simulink model "systema"  (Simulink 8.2)
settings: Solver=ode4  StartTime=0.0  StopTime=20  FixedStep=0.01  RelTol=1e-3
CloseFcn:
  | rtwprivate ssgencode ModelCloseRequest systema
settings Model: Creator=Administrator  LastModifiedBy=adnanmartini  BufferReuse=off
settings DataIOCC: SignalLoggingName=sigsOut
settings OptimizationCC: OptimizeBlockIOStorage=off  BufferReuse=off  ExpressionFolding=off  ExpressionDepthLimit=128  FoldNonRolledExpr=off  LocalBlockOutputs=off  InitFltsAndDblsToZero=on
settings DebuggingCC: SaveWithParameterizedLinksMsg=none  SignalResolutionControl=TryResolveAllWithWarning  SolverPrmCheckMsg=none  MultiTaskDSMMsg=warning  MultiTaskCondExecSysMsg=none
settings HardwareCC: TargetUnknown=on
settings SFSimCC: SimParseCustomCode=off
settings RTWCC: IncludeERTFirstTime=on
settings CodeAppCC: IgnoreCustomStorageClasses=off
settings GRTTargetCC: TargetFcnLib=ansi_tfl_tmw.mat  ModelReferenceCompliant=off  MatFileLogging=off

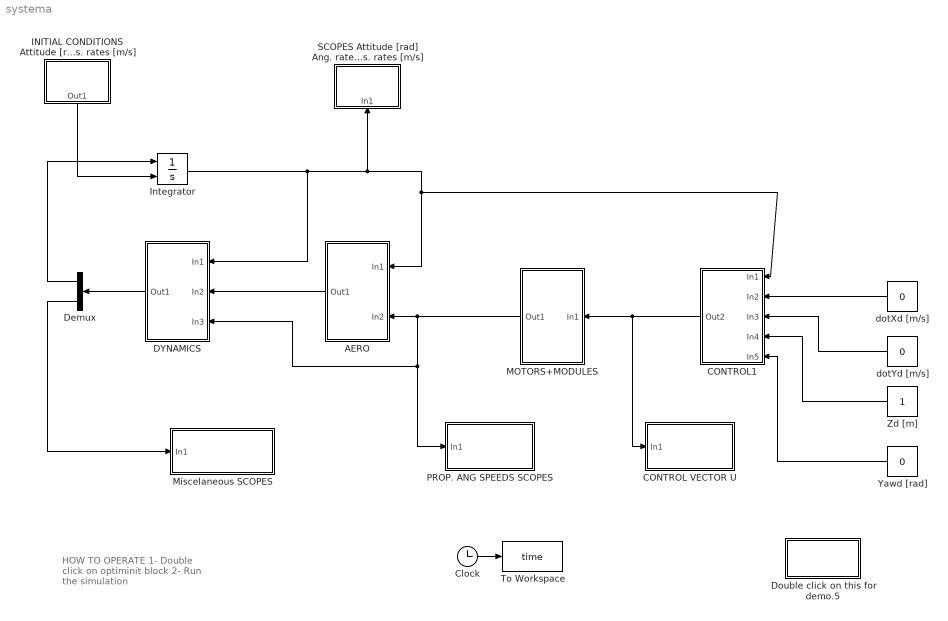
== system systema ==
  note: HOW TO OPERATE
      | 1- Double click on optiminit block
      | 2- Run the simulation
  AERO : Subsystem
  CONTROL VECTOR U : Subsystem
  CONTROL1 : Subsystem
  Clock : Clock
  DYNAMICS : Subsystem
  Demux : Demux  Outputs=2
  Double click on this for demo.5 : Subsystem
      settings: OpenFcn=optsiminit
      mask Display: disp('optsiminit')
  "INITIAL CONDITIONS Attitude [rad] Ang. rates [rad/sec] position [m] Pos. rates [m/s] " : Subsystem
  Integrator : Integrator  InitialConditionSource=external
  MOTORS+MODULES : Subsystem
  Miscelaneous SCOPES : Subsystem
  PROP. ANG SPEEDS SCOPES : Subsystem
  SCOPES Attitude [rad] Ang. rates [rad/sec] position [m] Pos. rates [m/s] : Subsystem
  To Workspace : ToWorkspace  VariableName=time  SampleTime=-1
  Yawd [rad] : Constant  Value=0
  Zd [m] : Constant
  dotXd [m/s] : Constant  Value=0
  dotYd [m/s] : Constant  Value=0
  wires:
  "INITIAL CONDITIONS Attitude [rad] Ang. rates [rad/sec] position [m] Pos. rates [m/s] "/1(Out1) -> Integrator/2
  Clock/1 -> To Workspace/1
  DYNAMICS/1(Out1) -> Demux/1
  Demux/1 -> Integrator/1
  Demux/2 -> Miscelaneous SCOPES/1(In1)
  CONTROL1/1(Out2) -> CONTROL VECTOR U/1(In1), MOTORS+MODULES/1(In1)
  dotXd [m/s]/1 -> CONTROL1/2(In2)
  dotYd [m/s]/1 -> CONTROL1/3(In3)
  Zd [m]/1 -> CONTROL1/4(In4)
  Yawd [rad]/1 -> CONTROL1/5(In5)
  MOTORS+MODULES/1(Out1) -> AERO/2(In2), DYNAMICS/3(In3), PROP. ANG SPEEDS SCOPES/1(In1)
  AERO/1(Out1) -> DYNAMICS/2(In2)
  Integrator/1 -> DYNAMICS/1(In1), CONTROL1/1(In1), AERO/1(In1), SCOPES Attitude [rad] Ang. rates [rad/sec] position [m] Pos. rates [m/s]/1(In1)

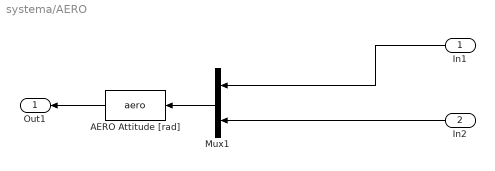
== system systema/AERO ==
  In1 : Inport
  In2 : Inport  Port=2
  AERO Attitude [rad] : MATLABFcn  MATLABFcn=aero  OutputDimensions=24
  Mux1 : Mux  Inputs=2
  Out1 : Outport
  wires:
  In1/1 -> Mux1/1
  In2/1 -> Mux1/2
  Mux1/1 -> AERO Attitude [rad]/1
  AERO Attitude [rad]/1 -> Out1/1

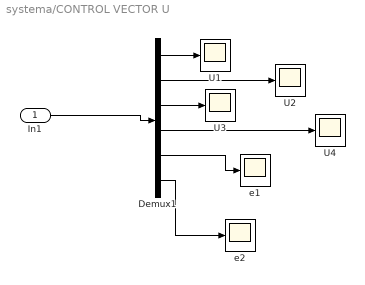
== system systema/CONTROL VECTOR U ==
  In1 : Inport
  Demux1 : Demux  Outputs=6
  U{1..4} (4 alike) : Scope
      U1 settings: TimeRange=3.5  YMin=4.25  YMax=9.75  SaveName=ScopeData7
      U2 settings: YMin=-0.6  YMax=0.4  SaveName=ScopeData8
      U3 settings: YMin=-0.65  YMax=0.35  SaveName=ScopeData9
      U4 settings: YMin=0  YMax=150  SaveName=ScopeData14
  e1 : Scope
      settings: YMin=0  YMax=150  SaveName=ScopeData11
  e2 : Scope
      settings: YMin=0  YMax=150  SaveName=ScopeData12
  wires:
  In1/1 -> Demux1/1
  Demux1/4 -> U4/1
  Demux1/3 -> U3/1
  Demux1/2 -> U2/1
  Demux1/1 -> U1/1
  Demux1/5 -> e1/1
  Demux1/6 -> e2/1

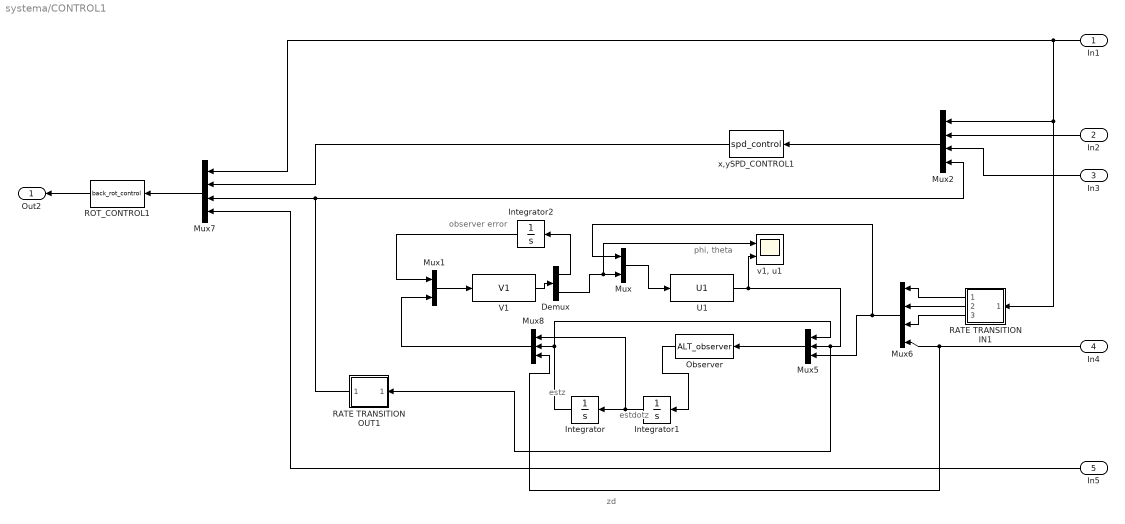
== system systema/CONTROL1 ==
  note: observer error
  note: phi, theta
  note: zd
  note: estz
  note: estdotz
  In1 : Inport
  In2 : Inport  Port=2
  In3 : Inport  Port=3
  In4 : Inport  Port=4
  In5 : Inport  Port=5
  Demux : Demux  Outputs=2
  Integrator : Integrator  InitialCondition=1
  Integrator1 : Integrator
  Integrator2 : Integrator
  Mux : Mux  Inputs=2
  Mux1 : Mux  Inputs=2
  Mux2 : Mux
  Mux5 : Mux  Inputs=3
  Mux6 : Mux
  Mux7 : Mux
  Mux8 : Mux  Inputs=3
  Observer : MATLABFcn  MATLABFcn=ALT_observer
  RATE TRANSITION IN1 : Subsystem
  RATE TRANSITION OUT1 : Subsystem
  ROT_CONTROL1 : MATLABFcn  MATLABFcn=back_rot_control  OutputDimensions=6
  U1 : MATLABFcn  MATLABFcn=U1  OutputDimensions=1
  V1 : MATLABFcn  MATLABFcn=V1  OutputDimensions=2
  "v1, u1" : Scope  NumInputPorts=2
      settings: TimeRange=20  YMin=-1.25~5.25  YMax=4.5~7.75  SaveName=ScopeData4
  x,ySPD_CONTROL1 : MATLABFcn  MATLABFcn=spd_control  OutputDimensions=2
  Out2 : Outport
  wires:
  Mux2/1 -> x,ySPD_CONTROL1/1
  ROT_CONTROL1/1 -> Out2/1
  In1/1 -> RATE TRANSITION IN1/1(In1), Mux2/1, Mux7/1
  In2/1 -> Mux2/2
  x,ySPD_CONTROL1/1 -> Mux7/2
  Mux7/1 -> ROT_CONTROL1/1
  In5/1 -> Mux7/4
  RATE TRANSITION OUT1/1(Out1) -> Mux2/4, Mux7/3
  RATE TRANSITION IN1/1(Out1) -> Mux6/1
  RATE TRANSITION IN1/2(Out2) -> Mux6/2
  RATE TRANSITION IN1/3(Out3) -> Mux6/3
  In4/1 -> Mux8/3, Mux6/4
  In3/1 -> Mux2/3
  Observer/1 -> Integrator1/1
  Mux6/1 -> Mux/1, Mux5/3
  Integrator1/1 -> Mux8/1, Integrator/1
  U1/1 -> RATE TRANSITION OUT1/1(In1), Mux5/2, "v1, u1"/2
  Mux5/1 -> Observer/1
  Integrator/1 -> Mux5/1, Mux8/2
  Mux/1 -> U1/1
  V1/1 -> Demux/1
  Demux/2 -> "v1, u1"/1, Mux/2
  Demux/1 -> Integrator2/1
  Mux1/1 -> V1/1
  Integrator2/1 -> Mux1/1
  Mux8/1 -> Mux1/2

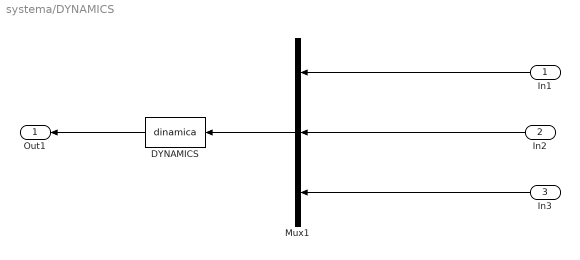
== system systema/DYNAMICS ==
  In1 : Inport
  In2 : Inport  Port=2
  In3 : Inport  Port=3
  DYNAMICS : MATLABFcn  MATLABFcn=dinamica  OutputDimensions=18
  Mux1 : Mux  Inputs=3
  Out1 : Outport
  wires:
  DYNAMICS/1 -> Out1/1
  Mux1/1 -> DYNAMICS/1
  In2/1 -> Mux1/2
  In1/1 -> Mux1/1
  In3/1 -> Mux1/3

== system systema/Double click on this for demo.5 ==

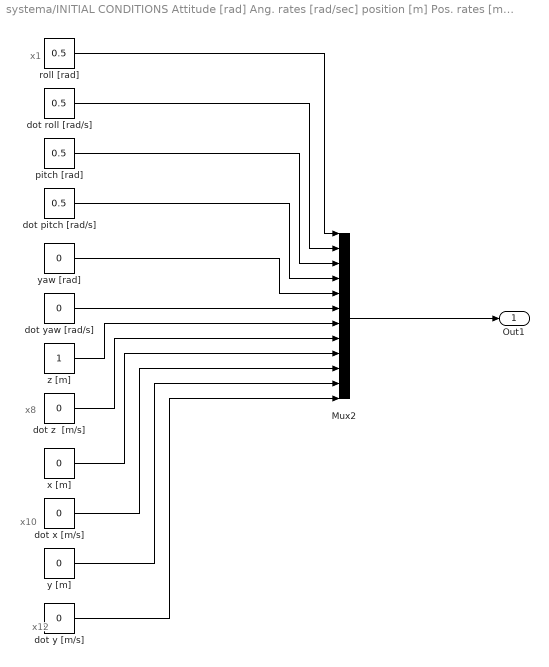
== system systema/INITIAL CONDITIONS Attitude [rad] Ang. rates [rad/sec] position [m] Pos. rates [m/s]  ==
  note: x1
  note: x12
  note: x10
  note: x8
  Mux2 : Mux  Inputs=12
  dot pitch [rad/s] : Constant  Value=0.5
  dot roll [rad/s] : Constant  Value=0.5
  dot x [m/s] : Constant  Value=0
  dot y [m/s] : Constant  Value=0
  dot yaw [rad/s] : Constant  Value=0
  dot z  [m/s] : Constant  Value=0
  pitch [rad] : Constant  Value=0.5
  roll [rad] : Constant  Value=0.5
  x [m] : Constant  Value=0
  y [m] : Constant  Value=0
  yaw [rad] : Constant  Value=0
  z [m] : Constant
  Out1 : Outport
  wires:
  roll [rad]/1 -> Mux2/1
  dot roll [rad/s]/1 -> Mux2/2
  pitch [rad]/1 -> Mux2/3
  dot pitch [rad/s]/1 -> Mux2/4
  dot yaw [rad/s]/1 -> Mux2/6
  z [m]/1 -> Mux2/7
  dot z  [m/s]/1 -> Mux2/8
  yaw [rad]/1 -> Mux2/5
  Mux2/1 -> Out1/1
  x [m]/1 -> Mux2/9
  dot x [m/s]/1 -> Mux2/10
  y [m]/1 -> Mux2/11
  dot y [m/s]/1 -> Mux2/12

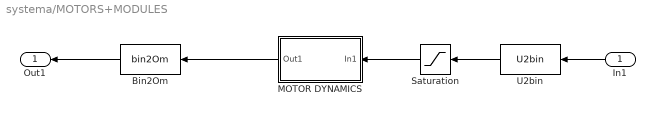
== system systema/MOTORS+MODULES ==
  In1 : Inport
  Bin2Om : MATLABFcn  MATLABFcn=bin2Om  OutputDimensions=4  OutputSignalType=real
  MOTOR DYNAMICS : Subsystem
  Saturation : Saturate  UpperLimit=125  LowerLimit=10
  U2bin : MATLABFcn  MATLABFcn=U2bin  OutputDimensions=4  OutputSignalType=real
  Out1 : Outport
  wires:
  Bin2Om/1 -> Out1/1
  MOTOR DYNAMICS/1(Out1) -> Bin2Om/1
  U2bin/1 -> Saturation/1
  In1/1 -> U2bin/1
  Saturation/1 -> MOTOR DYNAMICS/1(In1)

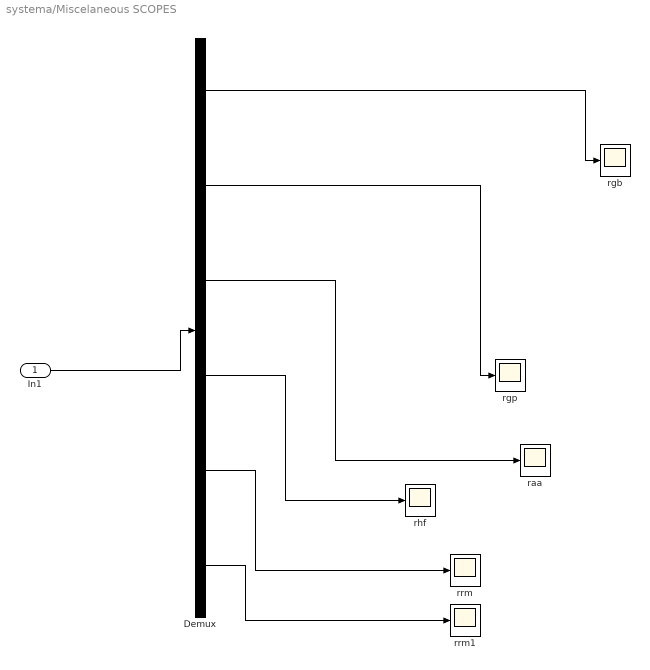
== system systema/Miscelaneous SCOPES ==
  In1 : Inport  PortDimensions=6
  Demux : Demux  Outputs=6
  raa : Scope
      settings: TimeRange=18  YMin=-200  YMax=200  SaveName=ScopeData16
  rgb : Scope
      settings: YMin=-0.25  YMax=-0.05  SaveName=ScopeData14
  rgp : Scope
      settings: YMin=-2250  YMax=2250  SaveName=ScopeData15
  rhf : Scope
      settings: TimeRange=10  YMin=-110.5  YMax=-107.25  SaveName=ScopeData18
  rrm : Scope
      settings: TimeRange=5  YMin=-4.75e-015  YMax=0  SaveName=ScopeData25
  rrm1 : Scope
      settings: TimeRange=5  YMin=-4.75e-015  YMax=0  SaveName=ScopeData3
  wires:
  In1/1 -> Demux/1
  Demux/5 -> rrm/1
  Demux/4 -> rhf/1
  Demux/3 -> raa/1
  Demux/2 -> rgp/1
  Demux/1 -> rgb/1
  Demux/6 -> rrm1/1

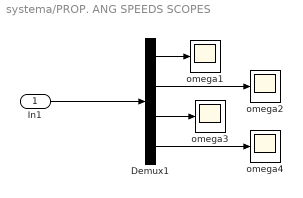
== system systema/PROP. ANG SPEEDS SCOPES ==
  In1 : Inport
  Demux1 : Demux
  omega{1..4} (4 alike) : Scope
      omega1 settings: TimeRange=3.5  YMin=144.101  YMax=144.104  SaveName=ScopeData7
      omega2 settings: YMin=142.5  YMax=147.5  SaveName=ScopeData8
      omega3 settings: YMin=0  YMax=150  SaveName=ScopeData9
      omega4 settings: YMin=0  YMax=150  SaveName=ScopeData14
  wires:
  Demux1/1 -> omega1/1
  Demux1/2 -> omega2/1
  Demux1/3 -> omega3/1
  Demux1/4 -> omega4/1
  In1/1 -> Demux1/1

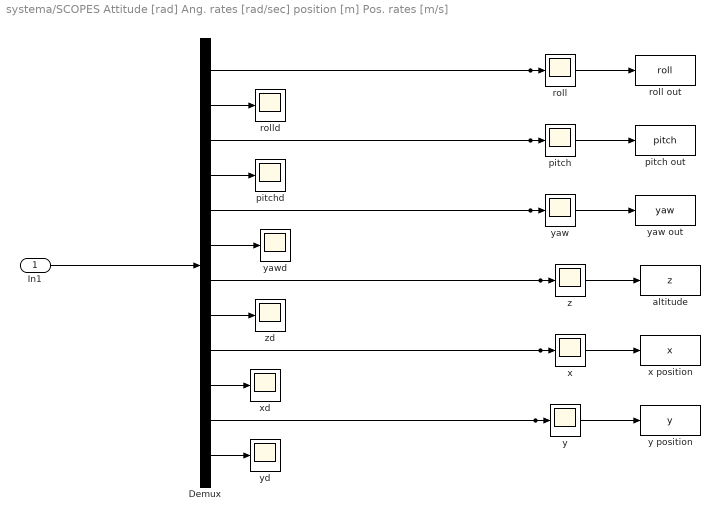
== system systema/SCOPES Attitude [rad] Ang. rates [rad/sec] position [m] Pos. rates [m/s] ==
  In1 : Inport
  Demux : Demux  Outputs=12
  altitude : ToWorkspace  VariableName=z  SampleTime=-1
  pitch : Scope
      settings: TimeRange=4  YMin=-0.08  YMax=0.16
  pitch out : ToWorkspace  VariableName=pitch  SampleTime=-1
  pitchd : Scope
      settings: YMin=-1.75  YMax=1.75  SaveName=ScopeData15
  roll : Scope
      settings: TimeRange=0.25  YMin=-0.008  YMax=0.005
  roll out : ToWorkspace  VariableName=roll  SampleTime=-1
  rolld : Scope
      settings: TimeRange=7  YMin=-0.15  YMax=0.125  SaveName=ScopeData14
  x : Scope
      settings: TimeRange=5  YMin=-1  YMax=1  SaveName=ScopeData24
  x position : ToWorkspace  VariableName=x  SampleTime=-1
  xd : Scope
      settings: TimeRange=5  YMin=-4.75e-015  YMax=0  SaveName=ScopeData25
  y : Scope
      settings: TimeRange=5  YMin=-1  YMax=1  SaveName=ScopeData26
  y position : ToWorkspace  VariableName=y  SampleTime=-1
  yaw : Scope
      settings: TimeRange=5  YMin=-175  YMax=0  SaveName=ScopeData2
  yaw out : ToWorkspace  VariableName=yaw  SampleTime=-1
  yawd : Scope
      settings: TimeRange=18  YMin=-0.275  YMax=0.15  SaveName=ScopeData16
  yd : Scope
      settings: TimeRange=5  YMin=-143.75  YMax=-141.75  SaveName=ScopeData27
  z : Scope
      settings: TimeRange=5  YMin=0  YMax=0.009  SaveName=ScopeData17
  zd : Scope
      settings: TimeRange=10  YMin=-110.5  YMax=-107.25  SaveName=ScopeData18
  wires:
  In1/1 -> Demux/1
  Demux/3 -> pitch/1, pitch out/1
  Demux/5 -> yaw/1, yaw out/1
  Demux/2 -> rolld/1
  Demux/6 -> yawd/1
  Demux/7 -> z/1, altitude/1
  Demux/8 -> zd/1
  Demux/9 -> x/1, x position/1
  Demux/11 -> y/1, y position/1
  Demux/12 -> yd/1
  Demux/10 -> xd/1
  Demux/4 -> pitchd/1
  Demux/1 -> roll/1, roll out/1

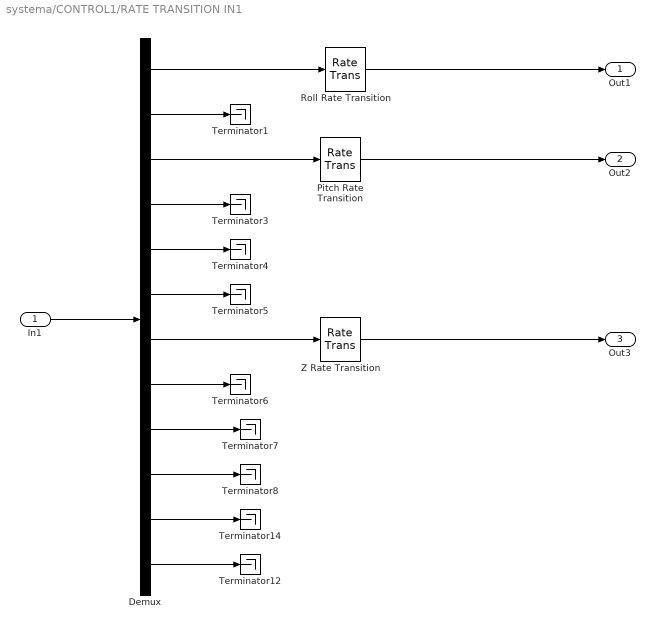
== system systema/CONTROL1/RATE TRANSITION IN1 ==
  In1 : Inport
  Demux : Demux  Outputs=12
  Pitch Rate Transition : RateTransition  Deterministic=off
  Roll Rate Transition : RateTransition  Deterministic=off
  Terminator{1,3..8,12,14} (9 alike) : Terminator
  Z Rate Transition : RateTransition  Deterministic=off
  Out1 : Outport
  Out2 : Outport  Port=2
  Out3 : Outport  Port=3
  wires:
  Demux/7 -> Z Rate Transition/1
  In1/1 -> Demux/1
  Demux/1 -> Roll Rate Transition/1
  Demux/2 -> Terminator1/1
  Demux/3 -> Pitch Rate Transition/1
  Demux/4 -> Terminator3/1
  Demux/5 -> Terminator4/1
  Demux/6 -> Terminator5/1
  Demux/9 -> Terminator7/1
  Demux/10 -> Terminator8/1
  Demux/11 -> Terminator14/1
  Demux/12 -> Terminator12/1
  Demux/8 -> Terminator6/1
  Roll Rate Transition/1 -> Out1/1
  Pitch Rate Transition/1 -> Out2/1
  Z Rate Transition/1 -> Out3/1

== system systema/CONTROL1/RATE TRANSITION OUT1 ==
  In1 : Inport
  Rate Transition1 : RateTransition  Deterministic=off
  Out1 : Outport
  wires:
  In1/1 -> Rate Transition1/1
  Rate Transition1/1 -> Out1/1

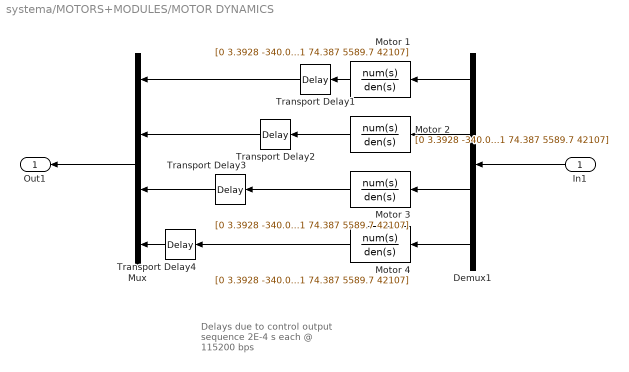
== system systema/MOTORS+MODULES/MOTOR DYNAMICS ==
  note: Delays due to control output sequence
      | 2E-4 s each @ 115200 bps
  In1 : Inport
  Demux1 : Demux
  Motor {1..4} (4 alike) : TransferFcn  Numerator=[0 3.3928 -340.09 39451]  Denominator=[1 74.387 5589.7 42107]
  Mux : Mux
  Transport Delay1 : TransportDelay  DelayTime=2E-4
  Transport Delay2 : TransportDelay  DelayTime=4E-4
  Transport Delay3 : TransportDelay  DelayTime=6E-4
  Transport Delay4 : TransportDelay  DelayTime=8E-4
  Out1 : Outport
  wires:
  In1/1 -> Demux1/1
  Demux1/1 -> Motor 1/1
  Demux1/2 -> Motor 2/1
  Demux1/3 -> Motor 3/1
  Demux1/4 -> Motor 4/1
  Motor 1/1 -> Transport Delay1/1
  Motor 2/1 -> Transport Delay2/1
  Motor 3/1 -> Transport Delay3/1
  Motor 4/1 -> Transport Delay4/1
  Mux/1 -> Out1/1
  Transport Delay2/1 -> Mux/2
  Transport Delay3/1 -> Mux/3
  Transport Delay4/1 -> Mux/4
  Transport Delay1/1 -> Mux/1
